simulink model "px4_6dof_quadrotor_bus"  (R2021b)
settings: Solver=VariableStepAuto  StartTime=0.0  StopTime=10.0  FixedStep=plant.motor.dynamic_time_sample/10  RelTol=1e-3
undefined symbols (not defined in the file or in its folder): angular_rate, ax, ay, az, body, controller, DiscIntNeverNeededParam, dphi, dpsi, dtheta, lag, land_detector, lead, magnitude, ned, notch, phi, pitch, plant, psi, rad, roll, s, theta, thrust, vx, vy, vz, w1, w2, w3, w4, x, y, yaw, z
libraries: cstblocks x33, aerolibconvert2 x4, simulink_extras x3, simulink x3, sharedtransform x1
(part 1 of 2)
settings Model: Creator=iftach  LastModifiedBy=iftach
settings SolverCC: ZeroCrossAlgorithm=Adaptive
settings DebuggingCC: MaskedZcDiagnostic=none  IgnoredZcDiagnostic=none

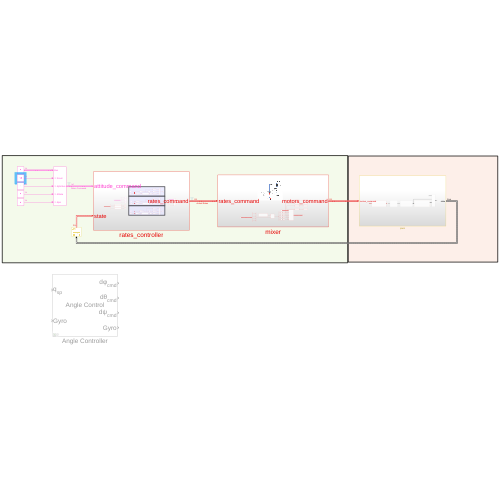
[thumbnail: Simulink's stored preview of the top-level diagram]
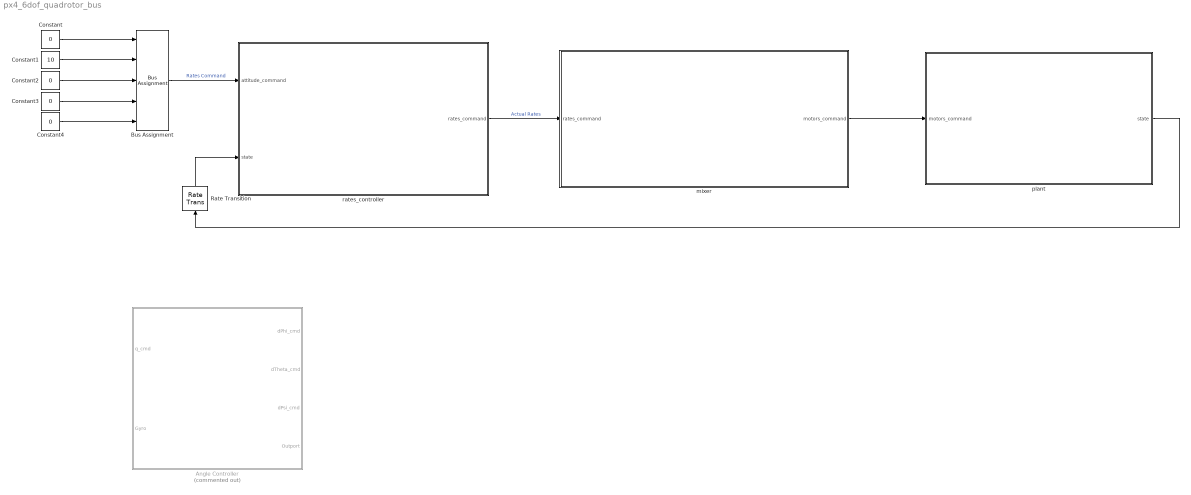
== system px4_6dof_quadrotor_bus ==
  Angle Controller : Subsystem  Commented=on  mask{MC_ROLL_P=4, MC_PITCH_P=4, MC_YAW_P=4, MC_ROLLRATE_MAX=2, MC_PITCHRATE_MAX=2, MC_YAWRATE_MAX=2, MC_ACRO_R_MAX=2, MC_YAW_WEIGHT=0.1, m=0.9}
      mask prompts: MC_ROLL_P "MC_ROLL_P ="; MC_PITCH_P "MC_PITCH_P ="; MC_YAW_P "MC_YAW_P ="; MC_ROLLRATE_MAX "MC_ROLLRATE_MAX ="; MC_PITCHRATE_MAX "MC_PITCHRATE_MAX ="; MC_YAWRATE_MAX "MC_YAWRATE_MAX ="; MC_ACRO_R_MAX "MC_ACRO_R_MAX ="; MC_YAW_WEIGHT "MC_YAW_WEIGHT ="; m "m [kg] ="
      mask DialogControl DescTextVar Prompt: Attitude Controller - based on PX4 architecture
      mask Display:
      | disp('Angle Control')
      | 
      | port_label('input',1,'q_{sp}','texmode','on')
      | port_label('input',2,'Gyro')
      | 
      | port_label('output',1,'d\phi_{cmd}','texmode','on')
      | port_label('output',2,'d\theta_{cmd}','texmode','on')
      | port_label('output',3,'d\psi_{cmd}','texmode','on')
      | port_label('output',4,'Gyro','texmode','on')
  Bus Assignment : BusAssignment  AssignedSignals=thrust,dphi,dtheta,dpsi
  Constant : Constant  Value=0  OutDataTypeStr=Bus: AttitudeCommand
  Constant1 : Constant  Value=10
  Constant2 : Constant  Value=0
  Constant3 : Constant  Value=0
  Constant4 : Constant  Value=0
  Rate Transition : RateTransition  OutPortSampleTime=controller.rate.time_sample
  mixer : Subsystem
  plant : Subsystem
  rates_controller : Subsystem
  wires:
  plant/1(state) -> Rate Transition/1
  mixer/1(motors_command) -> plant/1(motors_command)
  rates_controller/1(rates_command) -> mixer/1(rates_command)  "Actual Rates"
  Rate Transition/1 -> rates_controller/2(state)
  Constant/1 -> Bus Assignment/1
  Bus Assignment/1 -> rates_controller/1(attitude_command)  "Rates Command"
  Constant1/1 -> Bus Assignment/2
  Constant2/1 -> Bus Assignment/3
  Constant3/1 -> Bus Assignment/4
  Constant4/1 -> Bus Assignment/5

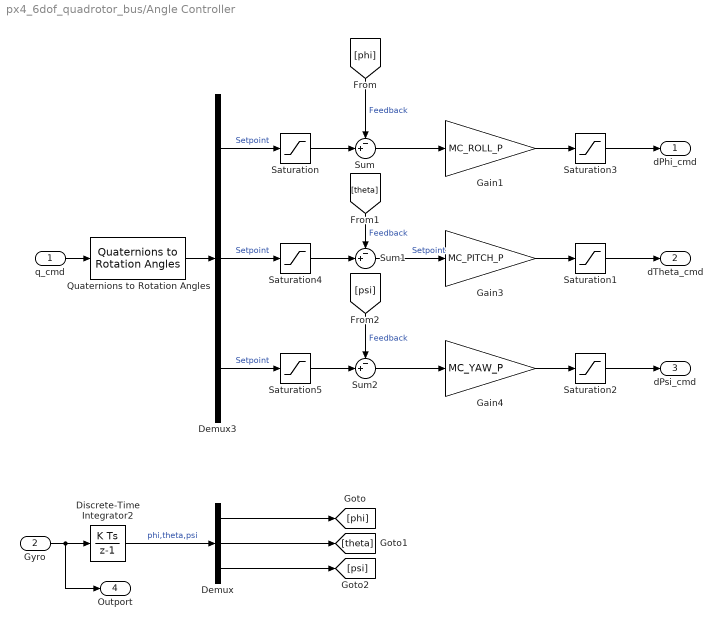
== system px4_6dof_quadrotor_bus/Angle Controller ==
  q_cmd : Inport
  Gyro : Inport  Port=2
  Demux : Demux  Outputs=3
  Demux3 : Demux  Outputs=3
  Discrete-Time Integrator2 : DiscreteIntegrator  InitialCondition=[0.001;0.001;0.001]  SampleTime=-1  ICPrevOutput=DiscIntNeverNeededParam  ICPrevScaledInput=DiscIntNeverNeededParam
  Gain1 : Gain  Gain=MC_ROLL_P
  Gain3 : Gain  Gain=MC_PITCH_P
  Gain4 : Gain  Gain=MC_YAW_P
  Quaternions to Rotation Angles : sharedtransform/Quaternions to Rotation Angles  rotationOrder=XYZ  aMode=aMode
      settings: SourceProductBaseCode=AE,PW,DR,MT,UV,VE
  Saturation : Saturate  UpperLimit=1.5  LowerLimit=-1.5
  Saturation1 : Saturate  UpperLimit=MC_PITCHRATE_MAX  LowerLimit=-MC_PITCHRATE_MAX
  Saturation2 : Saturate  UpperLimit=MC_YAWRATE_MAX  LowerLimit=-MC_YAWRATE_MAX
  Saturation3 : Saturate  UpperLimit=MC_ROLLRATE_MAX  LowerLimit=-MC_ROLLRATE_MAX
  Saturation4 : Saturate  UpperLimit=1.5  LowerLimit=-1.5
  Saturation5 : Saturate  UpperLimit=1.5  LowerLimit=-1.5
  Sum : Sum  Inputs=-+|
  Sum1 : Sum  Inputs=-+|
  Sum2 : Sum  Inputs=-+|
  dPhi_cmd : Outport
  dTheta_cmd : Outport  Port=2
  dPsi_cmd : Outport  Port=3
  Outport : Outport  Port=4
  wires:
  Saturation5/1 -> Sum2/2
  Saturation4/1 -> Sum1/2
  Saturation/1 -> Sum/2
  Quaternions to Rotation Angles/1 -> Demux3/1
  q_cmd/1 -> Quaternions to Rotation Angles/1
  Sum1/1 -> Gain3/1  "Setpoint"
  [psi] -> Sum2/1  "Feedback"
  Sum2/1 -> Gain4/1
  [theta] -> Sum1/1  "Feedback"
  Sum/1 -> Gain1/1
  [phi] -> Sum/1  "Feedback"
  Saturation2/1 -> dPsi_cmd/1
  Saturation1/1 -> dTheta_cmd/1
  Gain4/1 -> Saturation2/1
  Gain3/1 -> Saturation1/1
  Gain1/1 -> Saturation3/1
  Saturation3/1 -> dPhi_cmd/1
  Demux3/3 -> Saturation5/1  "Setpoint"
  Demux3/2 -> Saturation4/1  "Setpoint"
  Demux3/1 -> Saturation/1  "Setpoint"
  Demux/3 -> [psi]
  Demux/1 -> [phi]
  Demux/2 -> [theta]
  Gyro/1 -> Discrete-Time Integrator2/1, Outport/1
  Discrete-Time Integrator2/1 -> Demux/1  "phi,theta,psi"

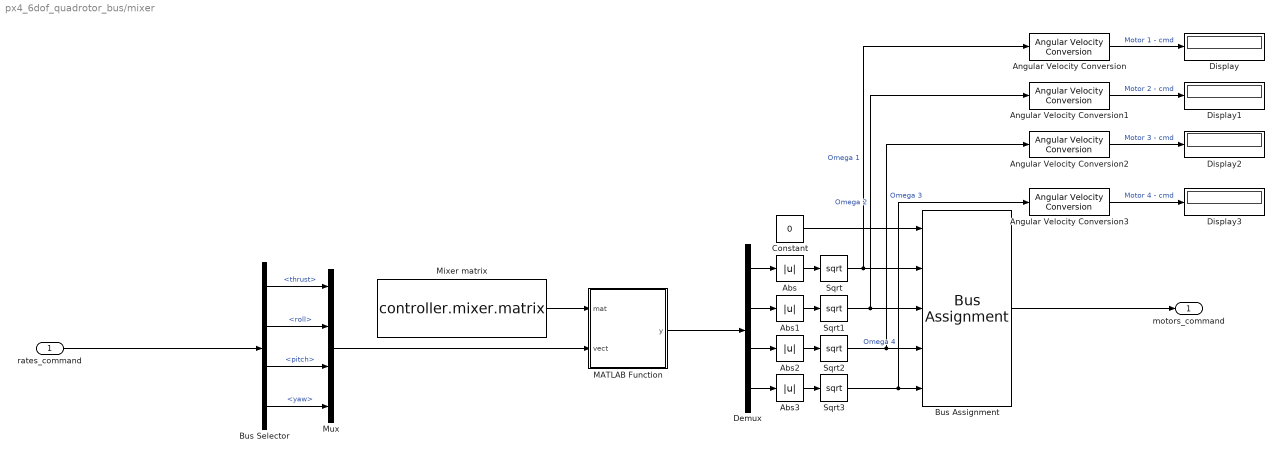
== system px4_6dof_quadrotor_bus/mixer ==
  rates_command : Inport  OutDataTypeStr=Bus: RatesCommand
  Abs{,1..3} (4 alike) : Abs
  Angular Velocity Conversion{,1..3} (4 alike) : aerolibconvert2/Angular Velocity Conversion  IU=rad/s  OU=rpm
  Bus Assignment : BusAssignment  AssignedSignals=w1,w2,w3,w4
  Bus Selector : BusSelector  OutputSignals=thrust,roll,pitch,yaw
  Constant : Constant  Value=0  OutDataTypeStr=Bus: MotorsCommand  SampleTime=controller.rate.time_sample
  Demux : Demux
  Display{,1..3} (4 alike) : Display
  MATLAB Function : MATLAB Function  TreatAsAtomicUnit=on
  Mixer matrix : Constant  StartFcn=|  Value=controller.mixer.matrix  OutDataTypeStr=Inherit: Inherit via back propagation  SampleTime=controller.rate.time_sample
      | %p = Simulink.Mask.get('ControlsModels/Moments and Forces');
      | 
      | Ct = 0.025
      | Cq = 2e-6;
      | 
      | %Ct = p.getParameter('Ct');
      | %Cq =p.getParameter('Cq');
      | 
      | %Ct = str2double(Ct.Value);
      | %Cq = str2double(Cq.Value);
  Mux : Mux
  Sqrt{,1..3} (4 alike) : Sqrt  SaturateOnIntegerOverflow=on
  motors_command : Outport
  wires:
  Demux/1 -> Abs/1
  Demux/2 -> Abs1/1
  Demux/3 -> Abs2/1
  Demux/4 -> Abs3/1
  MATLAB Function/1(y) -> Demux/1
  Mux/1 -> MATLAB Function/2(vect)
  Mixer matrix/1 -> MATLAB Function/1(mat)
  Sqrt/1 -> Bus Assignment/2, Angular Velocity Conversion/1  "Omega 1"
  Sqrt1/1 -> Bus Assignment/3, Angular Velocity Conversion1/1  "Omega 2"
  Sqrt2/1 -> Bus Assignment/4, Angular Velocity Conversion2/1  "Omega 3"
  Sqrt3/1 -> Bus Assignment/5, Angular Velocity Conversion3/1  "Omega 4"
  Angular Velocity Conversion/1 -> Display/1  "Motor 1 - cmd"
  Angular Velocity Conversion1/1 -> Display1/1  "Motor 2 - cmd"
  Angular Velocity Conversion2/1 -> Display2/1  "Motor 3 - cmd"
  Angular Velocity Conversion3/1 -> Display3/1  "Motor 4 - cmd"
  Abs/1 -> Sqrt/1
  Abs1/1 -> Sqrt1/1
  Abs2/1 -> Sqrt2/1
  Abs3/1 -> Sqrt3/1
  Constant/1 -> Bus Assignment/1
  Bus Assignment/1 -> motors_command/1
  rates_command/1 -> Bus Selector/1
  Bus Selector/1 -> Mux/1  "<thrust>"
  Bus Selector/2 -> Mux/2  "<roll>"
  Bus Selector/3 -> Mux/3  "<pitch>"
  Bus Selector/4 -> Mux/4  "<yaw>"

== system px4_6dof_quadrotor_bus/plant ==
  motors_command : Inport  OutDataTypeStr=Bus: MotorsCommand
  Bus Assignment : BusAssignment  AssignedSignals=body,ned,land_detector
  Constant : Constant  Value=0  OutDataTypeStr=Bus: PlantState  SampleTime=-1
  Rate Transition : RateTransition  OutPortSampleTime=0
  Rate Transition1 : RateTransition  OutPortSampleTime=0
  angle2body : Subsystem
  body2ned : Subsystem
  control2motors : Subsystem
  motors2angles : Subsystem
  state : Outport  OutDataTypeStr=Bus: PlantState
  wires:
  motors_command/1 -> control2motors/1(controller_command)
  control2motors/1(motors_velocities) -> Rate Transition/1  "Motors"
  motors2angles/1(angles) -> angle2body/1(angles)  "Body"
  angle2body/1(body) -> Bus Assignment/2, body2ned/1(body)
  Constant/1 -> Bus Assignment/1
  body2ned/1(NED) -> Bus Assignment/3
  Bus Assignment/1 -> state/1  "State"
  Rate Transition/1 -> motors2angles/1(motors_velocities)
  body2ned/2(land_detector) -> Rate Transition1/1
  Rate Transition1/1 -> Bus Assignment/4

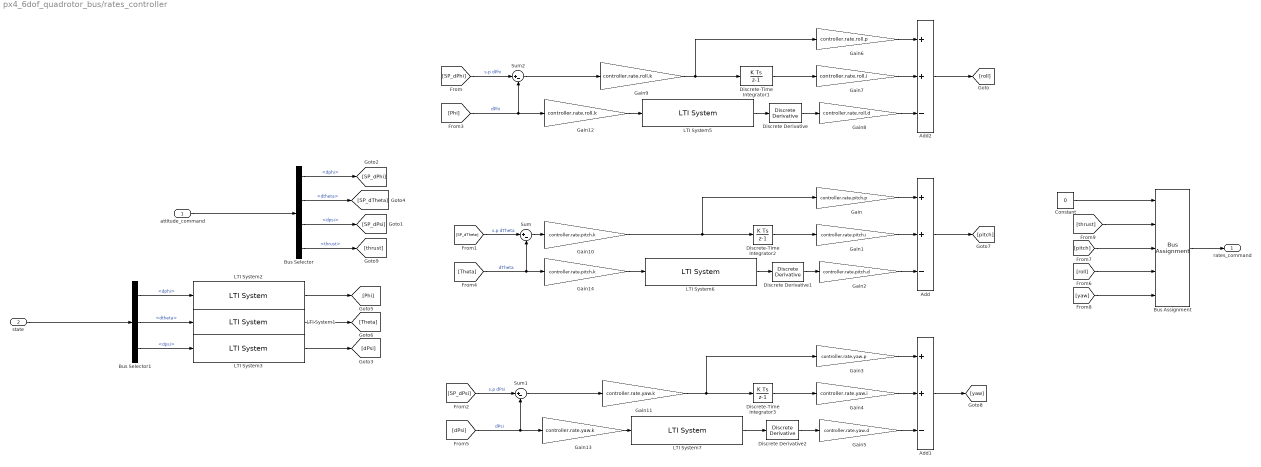
== system px4_6dof_quadrotor_bus/rates_controller ==
  attitude_command : Inport  OutDataTypeStr=Bus: AttitudeCommand
  state : Inport  Port=2  OutDataTypeStr=Bus: PlantState
  Add : Sum  Inputs=++-
  Add1 : Sum  Inputs=++-
  Add2 : Sum  Inputs=++-
  Bus Assignment : BusAssignment  AssignedSignals=thrust,pitch,roll,yaw
  Bus Selector : BusSelector  OutputSignals=dphi,dtheta,dpsi,thrust
  Bus Selector1 : BusSelector  OutputSignals=body.dphi,body.dtheta,body.dpsi
  Constant : Constant  Value=0  OutDataTypeStr=Bus: RatesCommand
  Discrete Derivative : simulink/Discrete/Discrete Derivative  gainval=1.0  ICPrevScaledInput=0.0  OutMin=[]  OutMax=[]  OutDataType=fixdt(1, 16)  OutScaling=2^-10  DoSatur=off
  Discrete Derivative1 : simulink/Discrete/Discrete Derivative  gainval=1.0  ICPrevScaledInput=0.0  OutMin=[]  OutMax=[]  OutDataType=fixdt(1, 16)  OutScaling=2^-10  DoSatur=off
  Discrete Derivative2 : simulink/Discrete/Discrete Derivative  gainval=1.0  ICPrevScaledInput=0.0  OutMin=[]  OutMax=[]  OutDataType=fixdt(1, 16)  OutScaling=2^-10  DoSatur=off
  Discrete-Time Integrator1 : DiscreteIntegrator  SampleTime=controller.rate.time_sample  LimitOutput=on  UpperSaturationLimit=controller.rate.mc_rr_int_limit  LowerSaturationLimit=-controller.rate.mc_rr_int_limit  ICPrevOutput=DiscIntNeverNeededParam  ICPrevScaledInput=DiscIntNeverNeededParam
  Discrete-Time Integrator2 : DiscreteIntegrator  SampleTime=controller.rate.time_sample  LimitOutput=on  UpperSaturationLimit=controller.rate.mc_pr_int_limit  LowerSaturationLimit=-controller.rate.mc_pr_int_limit  ICPrevOutput=DiscIntNeverNeededParam  ICPrevScaledInput=DiscIntNeverNeededParam
  Discrete-Time Integrator3 : DiscreteIntegrator  SampleTime=controller.rate.time_sample  LimitOutput=on  UpperSaturationLimit=controller.rate.mc_yr_int_limit  LowerSaturationLimit=-controller.rate.mc_yr_int_limit  ICPrevOutput=DiscIntNeverNeededParam  ICPrevScaledInput=DiscIntNeverNeededParam
  Gain : Gain  Gain=controller.rate.pitch.p
  Gain1 : Gain  Gain=controller.rate.pitch.i
  Gain10 : Gain  Gain=controller.rate.pitch.k
  Gain11 : Gain  Gain=controller.rate.yaw.k
  Gain12 : Gain  Gain=controller.rate.roll.k
  Gain13 : Gain  Gain=controller.rate.yaw.k
  Gain14 : Gain  Gain=controller.rate.pitch.k
  Gain2 : Gain  Gain=controller.rate.pitch.d
  Gain3 : Gain  Gain=controller.rate.yaw.p
  Gain4 : Gain  Gain=controller.rate.yaw.i
  Gain5 : Gain  Gain=controller.rate.yaw.d
  Gain6 : Gain  Gain=controller.rate.roll.p
  Gain7 : Gain  Gain=controller.rate.roll.i
  Gain8 : Gain  Gain=controller.rate.roll.d
  Gain9 : Gain  Gain=controller.rate.roll.k
  LTI System1 : cstblocks/LTI System  sys=c2d(tf(1,[controller.filters.gyro_cutoff 1]),controller.rate.time_sample)  IC=[]
  LTI System2 : cstblocks/LTI System  sys=c2d(tf(1,[controller.filters.gyro_cutoff 1]),controller.rate.time_sample)  IC=[]
  LTI System3 : cstblocks/LTI System  sys=c2d(tf(1,[controller.filters.gyro_cutoff 1]),controller.rate.time_sample)  IC=[]
  LTI System5 : cstblocks/LTI System  sys=c2d(tf(1,[controller.filters.dgyro_cutoff 1]),controller.rate.time_sample)  IC=[]
  LTI System6 : cstblocks/LTI System  sys=c2d(tf(1,[controller.filters.dgyro_cutoff 1]),controller.rate.time_sample)  IC=[]
  LTI System7 : cstblocks/LTI System  sys=c2d(tf(1,[controller.filters.dgyro_cutoff 1]),controller.rate.time_sample)  IC=[]
  Sum : Sum  Inputs=|+-
  Sum1 : Sum  Inputs=|+-
  Sum2 : Sum  Inputs=|+-
  rates_command : Outport  OutDataTypeStr=Bus: RatesCommand
  wires:
  Bus Selector/2 -> [SP_dTheta]  "<dtheta>"
  LTI System6/1 -> Discrete Derivative1/1
  Sum/1 -> Gain10/1
  Discrete-Time Integrator2/1 -> Gain1/1
  Gain2/1 -> Add/3
  Gain1/1 -> Add/2
  Gain/1 -> Add/1
  Gain3/1 -> Add1/1
  Gain4/1 -> Add1/2
  Gain5/1 -> Add1/3
  Discrete-Time Integrator3/1 -> Gain4/1
  Sum1/1 -> Gain11/1
  LTI System7/1 -> Discrete Derivative2/1
  [dPsi] -> Gain13/1, Sum1/2  "dPsi"
  [SP_dPsi] -> Sum1/1  "s.p dPsi"
  Add/1 -> [pitch]
  Bus Assignment/1 -> rates_command/1
  Gain6/1 -> Add2/1
  Gain7/1 -> Add2/2
  Gain8/1 -> Add2/3
  Discrete-Time Integrator1/1 -> Gain7/1
  Sum2/1 -> Gain9/1
  LTI System5/1 -> Discrete Derivative/1
  [SP_dPhi] -> Sum2/1  "s.p dPhi"
  [SP_dTheta] -> Sum/1  "s.p dTheta"
  [Phi] -> Gain12/1, Sum2/2  "dPhi"
  [Theta] -> Gain14/1, Sum/2  "dTheta"
  Add2/1 -> [roll]
  Add1/1 -> [yaw]
  Discrete Derivative/1 -> Gain8/1
  Discrete Derivative1/1 -> Gain2/1
  Discrete Derivative2/1 -> Gain5/1
  Gain9/1 -> Discrete-Time Integrator1/1, Gain6/1
  Gain10/1 -> Discrete-Time Integrator2/1, Gain/1
  Gain11/1 -> Discrete-Time Integrator3/1, Gain3/1
  Gain12/1 -> LTI System5/1
  Gain13/1 -> LTI System7/1
  Gain14/1 -> LTI System6/1
  state/1 -> Bus Selector1/1
  Bus Selector1/3 -> LTI System3/1  "<dpsi>"
  LTI System2/1 -> [Phi]
  LTI System1/1 -> [Theta]
  LTI System3/1 -> [dPsi]
  Bus Selector/3 -> [SP_dPsi]  "<dpsi>"
  Bus Selector/1 -> [SP_dPhi]  "<dphi>"
  attitude_command/1 -> Bus Selector/1
  Bus Selector1/1 -> LTI System2/1  "<dphi>"
  Bus Selector1/2 -> LTI System1/1  "<dtheta>"
  Constant/1 -> Bus Assignment/1
  [roll] -> Bus Assignment/4
  [pitch] -> Bus Assignment/3
  [yaw] -> Bus Assignment/5
  Bus Selector/4 -> [thrust]  "<thrust>"
  [thrust] -> Bus Assignment/2

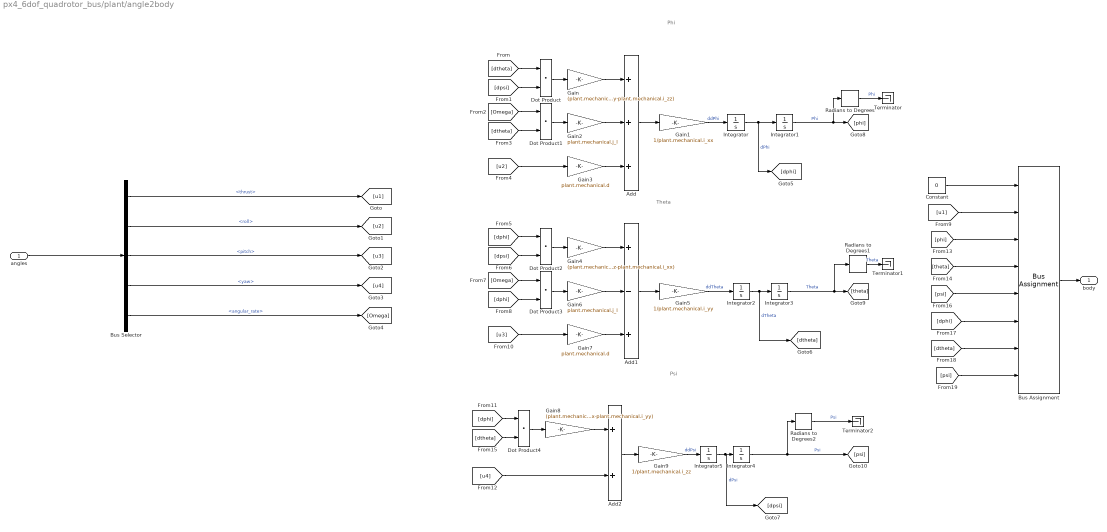
== system px4_6dof_quadrotor_bus/plant/angle2body ==
  note: Phi
  note: Theta
  note: Psi
  angles : Inport  OutDataTypeStr=Bus: PlantAngles
  Add : Sum  Inputs=3
  Add1 : Sum  Inputs=+-+
  Add2 : Sum  Inputs=2
  Bus Assignment : BusAssignment  AssignedSignals=thrust,phi,theta,psi,dphi,dtheta,dpsi
  Bus Selector : BusSelector  OutputSignals=thrust,roll,pitch,yaw,angular_rate
  Constant : Constant  Value=0  OutDataTypeStr=Bus: PlantBody  SampleTime=-1
  Dot Product{,1..4} (5 alike) : DotProduct  InputSameDT=on  OutDataTypeStr=Inherit: Inherit via internal rule
  Gain : Gain  Gain=(plant.mechanical.i_yy-plant.mechanical.i_zz)
  Gain1 : Gain  Gain=1/plant.mechanical.i_xx
  Gain2 : Gain  Gain=plant.mechanical.j_l
  Gain3 : Gain  Gain=plant.mechanical.d
  Gain4 : Gain  Gain=(plant.mechanical.i_zz-plant.mechanical.i_xx)
  Gain5 : Gain  Gain=1/plant.mechanical.i_yy
  Gain6 : Gain  Gain=plant.mechanical.j_l
  Gain7 : Gain  Gain=plant.mechanical.d
  Gain8 : Gain  Gain=(plant.mechanical.i_xx-plant.mechanical.i_yy)
  Gain9 : Gain  Gain=1/plant.mechanical.i_zz
  Integrator{,1..5} (6 alike) : Integrator
  Radians to Degrees : simulink_extras/Transformations/Radians to Degrees
  Radians to Degrees1 : simulink_extras/Transformations/Radians to Degrees
  Radians to Degrees2 : simulink_extras/Transformations/Radians to Degrees
  Terminator : Terminator
  Terminator1 : Terminator
  Terminator2 : Terminator
  body : Outport  OutDataTypeStr=Bus: PlantBody
  wires:
  Integrator/1 -> [dphi], Integrator1/1  "dPhi"
  Integrator2/1 -> Integrator3/1, [dtheta]  "dTheta"
  Integrator5/1 -> [dpsi], Integrator4/1  "dPsi"
  Integrator1/1 -> [phi], Radians to Degrees/1  "Phi"
  Integrator3/1 -> Radians to Degrees1/1, [theta]  "Theta"
  Integrator4/1 -> Radians to Degrees2/1, [psi]  "Psi"
  [dpsi] -> Dot Product/2
  [dtheta] -> Dot Product/1
  Dot Product/1 -> Gain/1
  Gain/1 -> Add/1
  Gain1/1 -> Integrator/1  "ddPhi"
  Add/1 -> Gain1/1
  [Omega] -> Dot Product1/1
  Dot Product1/1 -> Gain2/1
  [dtheta] -> Dot Product1/2
  Gain2/1 -> Add/2
  [u2] -> Gain3/1
  Gain7/1 -> Add1/3
  [u3] -> Gain7/1
  Gain6/1 -> Add1/2
  [dphi] -> Dot Product3/2
  Dot Product3/1 -> Gain6/1
  [Omega] -> Dot Product3/1
  Add1/1 -> Gain5/1
  Gain4/1 -> Add1/1
  Dot Product2/1 -> Gain4/1
  [dphi] -> Dot Product2/1
  [dpsi] -> Dot Product2/2
  Gain5/1 -> Integrator2/1  "ddTheta"
  [dtheta] -> Dot Product4/2
  Dot Product4/1 -> Gain8/1
  Gain8/1 -> Add2/1
  Add2/1 -> Gain9/1
  Gain9/1 -> Integrator5/1  "ddPsi"
  [dphi] -> Dot Product4/1
  [u4] -> Add2/2
  Gain3/1 -> Add/3
  Radians to Degrees/1 -> Terminator/1  "Phi"
  Radians to Degrees1/1 -> Terminator1/1  "Theta"
  Radians to Degrees2/1 -> Terminator2/1  "Psi"
  Bus Selector/1 -> [u1]  "<thrust>"
  Bus Selector/2 -> [u2]  "<roll>"
  Bus Selector/3 -> [u3]  "<pitch>"
  Bus Selector/4 -> [u4]  "<yaw>"
  Bus Selector/5 -> [Omega]  "<angular_rate>"
  Bus Assignment/1 -> body/1
  Constant/1 -> Bus Assignment/1
  [u1] -> Bus Assignment/2
  [phi] -> Bus Assignment/3
  [theta] -> Bus Assignment/4
  [psi] -> Bus Assignment/5
  [dphi] -> Bus Assignment/6
  [dtheta] -> Bus Assignment/7
  [psi] -> Bus Assignment/8
  angles/1 -> Bus Selector/1

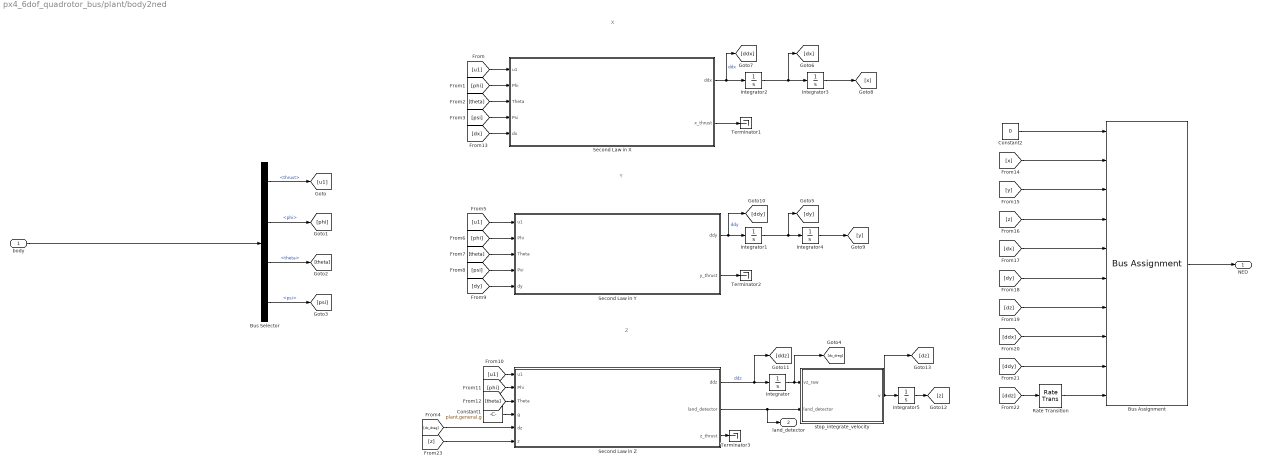
== system px4_6dof_quadrotor_bus/plant/body2ned ==
  note: X
  note: Y
  note: Z
  body : Inport  OutDataTypeStr=Bus: PlantBody
  Bus Assignment : BusAssignment  AssignedSignals=x,y,z,vx,vy,vz,ax,ay,az
  Bus Selector : BusSelector  OutputSignals=thrust,phi,theta,psi
  Constant1 : Constant  Value=plant.general.g  SampleTime=-1
  Constant2 : Constant  Value=0  OutDataTypeStr=Bus: PlantNed
  Integrator : Integrator  InitialCondition=plant.ic.velocity.z
  Integrator1 : Integrator  InitialCondition=plant.ic.velocity.y
  Integrator2 : Integrator  InitialCondition=plant.ic.velocity.x
  Integrator3 : Integrator  InitialCondition=plant.ic.position.x
  Integrator4 : Integrator  InitialCondition=plant.ic.position.y
  Integrator5 : Integrator  InitialCondition=plant.ic.position.z  LimitOutput=on  UpperSaturationLimit=0
  Rate Transition : RateTransition  OutPortSampleTime=0
  Second Law in X : Subsystem
  Second Law in Y : Subsystem
  Second Law in Z : Subsystem
  Terminator1 : Terminator
  Terminator2 : Terminator
  Terminator3 : Terminator
  stop_integrate_velocity : MATLAB Function  TreatAsAtomicUnit=on
  NED : Outport  OutDataTypeStr=Bus: PlantNed
  land_detector : Outport  Port=2  OutDataTypeStr=boolean
  wires:
  Second Law in X/1(ddx) -> [ddx], Integrator2/1  "ddx"
  [u1] -> Second Law in X/1(u1)
  [phi] -> Second Law in X/2(Phi)
  [theta] -> Second Law in X/3(Theta)
  [psi] -> Second Law in X/4(Psi)
  [psi] -> Second Law in Y/4(Psi)
  [theta] -> Second Law in Y/3(Theta)
  [phi] -> Second Law in Y/2(Phi)
  [u1] -> Second Law in Y/1(u1)
  Second Law in Y/1(ddy) -> [ddy], Integrator1/1  "ddy"
  Second Law in Z/1(ddz) -> Integrator/1, [ddz]  "ddz"
  [u1] -> Second Law in Z/1(u1)
  [phi] -> Second Law in Z/2(Phi)
  [theta] -> Second Law in Z/3(Theta)
  Constant1/1 -> Second Law in Z/4(g)
  [dy] -> Second Law in Y/5(dy)
  [dx] -> Second Law in X/5(dx)
  Integrator2/1 -> Integrator3/1, [dx]
  Integrator1/1 -> Integrator4/1, [dy]
  body/1 -> Bus Selector/1
  Bus Selector/1 -> [u1]  "<thrust>"
  Bus Selector/2 -> [phi]  "<phi>"
  Bus Selector/3 -> [theta]  "<theta>"
  Bus Selector/4 -> [psi]  "<psi>"
  Integrator3/1 -> [x]
  Integrator4/1 -> [y]
  Constant2/1 -> Bus Assignment/1
  [x] -> Bus Assignment/2
  [y] -> Bus Assignment/3
  [z] -> Bus Assignment/4
  [dx] -> Bus Assignment/5
  [dy] -> Bus Assignment/6
  [dz] -> Bus Assignment/7
  [ddx] -> Bus Assignment/8
  [ddy] -> Bus Assignment/9
  [ddz] -> Rate Transition/1
  Bus Assignment/1 -> NED/1
  Second Law in X/2(x_thrust) -> Terminator1/1
  Second Law in Y/2(y_thrust) -> Terminator2/1
  Second Law in Z/3(z_thrust) -> Terminator3/1
  Integrator5/1 -> [z]
  [dz_drag] -> Second Law in Z/5(dz)
  Second Law in Z/2(land_detector) -> land_detector/1, stop_integrate_velocity/2(land_detector)
  [z] -> Second Law in Z/6(z)
  Integrator/1 -> [dz_drag], stop_integrate_velocity/1(vz_raw)
  Rate Transition/1 -> Bus Assignment/10
  stop_integrate_velocity/1(v) -> [dz], Integrator5/1

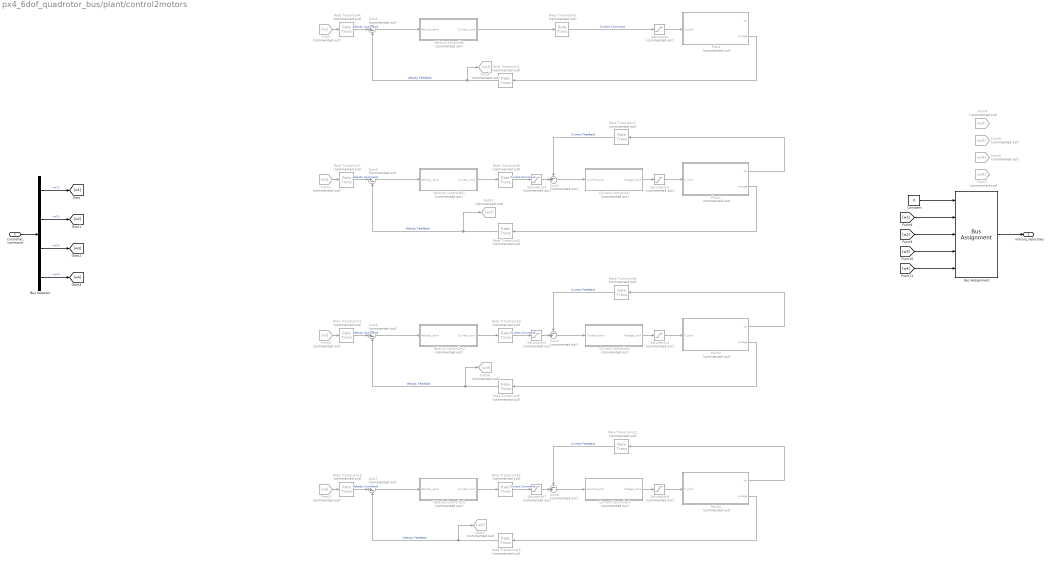
== system px4_6dof_quadrotor_bus/plant/control2motors ==
  controller_command : Inport  OutDataTypeStr=Bus: MotorsCommand
  Bus Assignment : BusAssignment  AssignedSignals=w1,w2,w3,w4
  Bus Selector : BusSelector  OutputSignals=w1,w2,w3,w4
  Constant : Constant  Value=0  OutDataTypeStr=Bus: PlantMotorsVelocity
  Current Controller1 : Subsystem  Commented=on
  Current Controller2 : Subsystem  Commented=on
  Current Controller3 : Subsystem  Commented=on
  From : From  Commented=on  GotoTag=w1
  From1 : From  Commented=on  GotoTag=w2
  From2 : From  Commented=on  GotoTag=w3
  From3 : From  Commented=on  GotoTag=w4
  From4 : From  Commented=on  GotoTag=w1f
  From5 : From  Commented=on  GotoTag=w2f
  From6 : From  Commented=on  GotoTag=w3f
  From7 : From  Commented=on  GotoTag=w4f
  Goto4 : Goto  Commented=on  GotoTag=w1f
  Goto5 : Goto  Commented=on  GotoTag=w2f
  Goto6 : Goto  Commented=on  GotoTag=w3f
  Goto7 : Goto  Commented=on  GotoTag=w4f
  Plant : Subsystem  Commented=on
  Plant1 : Subsystem  Commented=on
  Plant2 : Subsystem  Commented=on
  Plant3 : Subsystem  Commented=on
  Rate Transition{1,3,6,8,10,12,14} (7 alike) : RateTransition  Commented=on  OutPortSampleTime=plant.motor.electric_time_sample
  Rate Transition{2,4..5,7,9,11,13,15} (8 alike) : RateTransition  Commented=on  OutPortSampleTime=plant.motor.dynamic_time_sample
  Saturation{,1,4,6} (4 alike) : Saturate  Commented=on  UpperLimit=plant.motor.max_v  LowerLimit=-plant.motor.max_v
  Saturation3 : Saturate  Commented=on  UpperLimit=plant.motor.max_i  LowerLimit=-plant.motor.max_i
  Saturation5 : Saturate  Commented=on  UpperLimit=plant.motor.max_i  LowerLimit=-plant.motor.max_i
  Saturation7 : Saturate  Commented=on  UpperLimit=plant.motor.max_i  LowerLimit=-plant.motor.max_i
  Sum{1,3,5,7} (4 alike) : Sum  Commented=on  Inputs=|+-
  Sum2 : Sum  Commented=on  Inputs=-+|
  Sum4 : Sum  Commented=on  Inputs=-+|
  Sum6 : Sum  Commented=on  Inputs=-+|
  Velocity Controller : Subsystem  Commented=on
  Velocity Controller1 : Subsystem  Commented=on
  Velocity Controller2 : Subsystem  Commented=on
  Velocity Controller3 : Subsystem  Commented=on
  motors_velocities : Outport  OutDataTypeStr=Bus: PlantMotorsVelocity
  wires:
  Saturation/1 -> Plant/1(V_cmd)
  Velocity Controller/1(Current_cmd) -> Rate Transition3/1
  Rate Transition3/1 -> Saturation/1  "Current Command"
  Rate Transition2/1 -> Goto4/1, Sum1/2  "Velocity Feedback"
  Plant/2(omega) -> Rate Transition2/1
  Sum1/1 -> Velocity Controller/1(Velocity_error)
  Rate Transition4/1 -> Sum1/1  "Velocity Command"
  Rate Transition7/1 -> Sum3/1  "Velocity Command"
  Sum2/1 -> Current Controller1/1(Current_error)
  Saturation1/1 -> Plant1/1(V_cmd)
  Rate Transition1/1 -> Sum2/1  "Current Feedback"
  Sum3/1 -> Velocity Controller1/1(Velocity_error)
  Current Controller1/1(Voltage_cmd) -> Saturation1/1
  Plant1/2(omega) -> Rate Transition5/1
  Saturation3/1 -> Sum2/2
  Plant1/1(Im) -> Rate Transition1/1
  Rate Transition5/1 -> Goto5/1, Sum3/2  "Velocity Feedback"
  Rate Transition6/1 -> Saturation3/1  "Current Command"
  Velocity Controller1/1(Current_cmd) -> Rate Transition6/1
  Rate Transition11/1 -> Sum5/1  "Velocity Command"
  Sum4/1 -> Current Controller2/1(Current_error)
  Saturation4/1 -> Plant2/1(V_cmd)
  Rate Transition8/1 -> Sum4/1  "Current Feedback"
  Sum5/1 -> Velocity Controller2/1(Velocity_error)
  Current Controller2/1(Voltage_cmd) -> Saturation4/1
  Plant2/2(omega) -> Rate Transition9/1
  Saturation5/1 -> Sum4/2
  Plant2/1(Im) -> Rate Transition8/1
  Rate Transition9/1 -> Goto6/1, Sum5/2  "Velocity Feedback"
  Rate Transition10/1 -> Saturation5/1  "Current Command"
  Velocity Controller2/1(Current_cmd) -> Rate Transition10/1
  Rate Transition15/1 -> Sum7/1  "Velocity Command"
  Sum6/1 -> Current Controller3/1(Current_error)
  Saturation6/1 -> Plant3/1(V_cmd)
  Rate Transition12/1 -> Sum6/1  "Current Feedback"
  Sum7/1 -> Velocity Controller3/1(Velocity_error)
  Current Controller3/1(Voltage_cmd) -> Saturation6/1
  Plant3/2(omega) -> Rate Transition13/1
  Saturation7/1 -> Sum6/2
  Plant3/1(Im) -> Rate Transition12/1
  Rate Transition13/1 -> Goto7/1, Sum7/2  "Velocity Feedback"
  Rate Transition14/1 -> Saturation7/1  "Current Command"
  Velocity Controller3/1(Current_cmd) -> Rate Transition14/1
  controller_command/1 -> Bus Selector/1
  Bus Selector/1 -> [w1]  "<w1>"
  Bus Selector/2 -> [w2]  "<w2>"
  Bus Selector/3 -> [w3]  "<w3>"
  Bus Selector/4 -> [w4]  "<w4>"
  From/1 -> Rate Transition4/1
  From1/1 -> Rate Transition7/1
  From2/1 -> Rate Transition11/1
  From3/1 -> Rate Transition15/1
  Constant/1 -> Bus Assignment/1
  [w1] -> Bus Assignment/2
  [w2] -> Bus Assignment/3
  [w3] -> Bus Assignment/4
  [w4] -> Bus Assignment/5
  Bus Assignment/1 -> motors_velocities/1

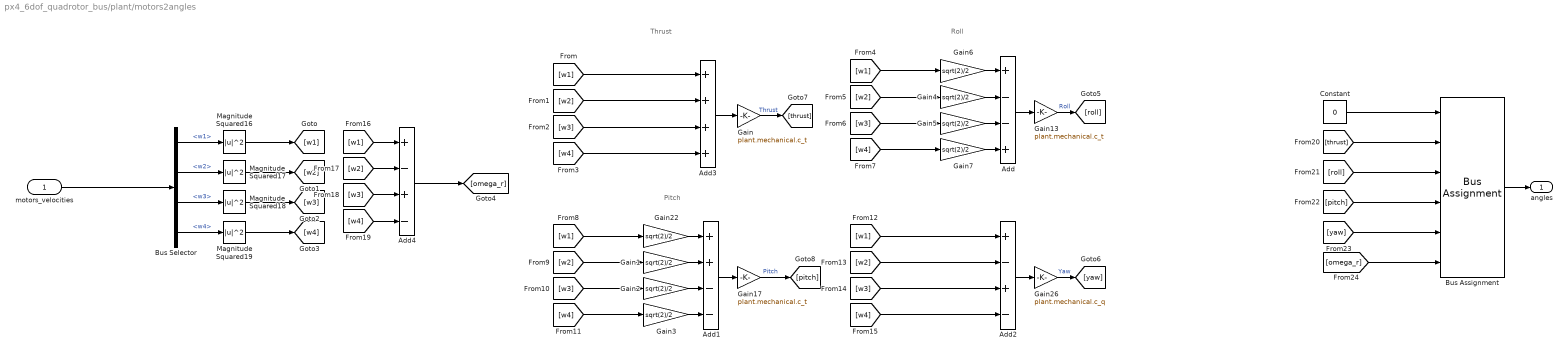
== system px4_6dof_quadrotor_bus/plant/motors2angles ==
  note: Thrust
  note: Roll
  note: Pitch
  motors_velocities : Inport  OutDataTypeStr=Bus: PlantMotorsVelocity
  Add : Sum  Inputs=+--+
  Add1 : Sum  Inputs=++--
  Add2 : Sum  Inputs=+-+-
  Add3 : Sum  Inputs=4
  Add4 : Sum  Inputs=+-+-
  Bus Assignment : BusAssignment  AssignedSignals=thrust,roll,pitch,yaw,angular_rate
  Bus Selector : BusSelector  OutputSignals=w1,w2,w3,w4
  Constant : Constant  Value=0  OutDataTypeStr=Bus: PlantAngles
  Gain : Gain  Gain=plant.mechanical.c_t
  Gain{1..7,22} (8 alike) : Gain  Gain=sqrt(2)/2
  Gain13 : Gain  Gain=plant.mechanical.c_t
  Gain17 : Gain  Gain=plant.mechanical.c_t
  Gain26 : Gain  Gain=plant.mechanical.c_q
  Magnitude Squared{16..19} (4 alike) : Math  Operator=magnitude^2  SaturateOnIntegerOverflow=on
  angles : Outport  OutDataTypeStr=Bus: PlantAngles
  wires:
  [w2] -> Gain4/1
  Gain/1 -> [thrust]  "Thrust"
  Gain1/1 -> Add1/2
  [w3] -> Add2/3
  [w3] -> Gain5/1
  [w3] -> Gain2/1
  Gain22/1 -> Add1/1
  Gain6/1 -> Add/1
  [w1] -> Gain6/1
  Gain2/1 -> Add1/3
  [w4] -> Add2/4
  [w1] -> Gain22/1
  Bus Selector/1 -> Magnitude Squared16/1  "<w1>"
  Bus Selector/2 -> Magnitude Squared17/1  "<w2>"
  Gain13/1 -> [roll]  "Roll"
  Add1/1 -> Gain17/1
  [w1] -> Add2/1
  [w3] -> Add3/3
  [w2] -> Add3/2
  [w2] -> Add4/2
  Gain4/1 -> Add/2
  Bus Selector/4 -> Magnitude Squared19/1  "<w4>"
  Gain26/1 -> [yaw]  "Yaw"
  [w4] -> Gain7/1
  [w2] -> Add2/2
  Bus Selector/3 -> Magnitude Squared18/1  "<w3>"
  Gain3/1 -> Add1/4
  Add/1 -> Gain13/1
  Add3/1 -> Gain/1
  Add2/1 -> Gain26/1
  [w4] -> Add4/4
  [w4] -> Add3/4
  [w1] -> Add3/1
  [w2] -> Gain1/1
  [w4] -> Gain3/1
  Gain5/1 -> Add/3
  Gain7/1 -> Add/4
  [w1] -> Add4/1
  [w3] -> Add4/3
  Gain17/1 -> [pitch]  "Pitch"
  Add4/1 -> [omega_r]
  Bus Assignment/1 -> angles/1
  Constant/1 -> Bus Assignment/1
  motors_velocities/1 -> Bus Selector/1
  [thrust] -> Bus Assignment/2
  [roll] -> Bus Assignment/3
  [pitch] -> Bus Assignment/4
  [yaw] -> Bus Assignment/5
  [omega_r] -> Bus Assignment/6
  Magnitude Squared16/1 -> [w1]
  Magnitude Squared17/1 -> [w2]
  Magnitude Squared18/1 -> [w3]
  Magnitude Squared19/1 -> [w4]

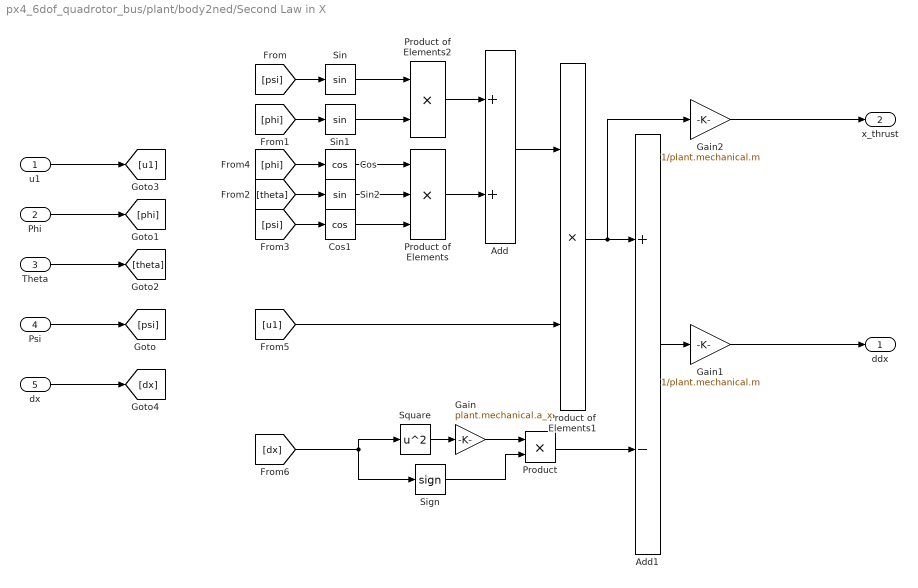
== system px4_6dof_quadrotor_bus/plant/body2ned/Second Law in X ==
  u1 : Inport
  Phi : Inport  Port=2
  Theta : Inport  Port=3
  Psi : Inport  Port=4
  dx : Inport  Port=5
  Add : Sum
  Add1 : Sum  Inputs=+-
  Cos : Trigonometry  Operator=cos
  Cos1 : Trigonometry  Operator=cos
  Gain : Gain  Gain=plant.mechanical.a_x
  Gain1 : Gain  Gain=1/plant.mechanical.m
  Gain2 : Gain  Gain=1/plant.mechanical.m
  Product : Product
  Product of Elements : Product  Inputs=3
  Product of Elements1 : Product
  Product of Elements2 : Product
  Sign : Signum
  Sin : Trigonometry
  Sin1 : Trigonometry
  Sin2 : Trigonometry
  Square : Math  Operator=square  SaturateOnIntegerOverflow=on
  ddx : Outport
  x_thrust : Outport  Port=2
  wires:
  Cos/1 -> Product of Elements/1
  [phi] -> Cos/1
  [psi] -> Cos1/1
  Cos1/1 -> Product of Elements/3
  Sin1/1 -> Product of Elements2/2
  [u1] -> Product of Elements1/2
  Product of Elements/1 -> Add/2
  Product of Elements1/1 -> Gain2/1, Add1/1
  Add/1 -> Product of Elements1/1
  [theta] -> Sin2/1
  Sin2/1 -> Product of Elements/2
  Product of Elements2/1 -> Add/1
  [psi] -> Sin/1
  Sin/1 -> Product of Elements2/1
  [phi] -> Sin1/1
  Add1/1 -> Gain1/1
  Psi/1 -> [psi]
  Phi/1 -> [phi]
  Theta/1 -> [theta]
  u1/1 -> [u1]
  dx/1 -> [dx]
  Gain1/1 -> ddx/1
  Square/1 -> Gain/1
  [dx] -> Square/1, Sign/1
  Gain/1 -> Product/1
  Sign/1 -> Product/2
  Product/1 -> Add1/2
  Gain2/1 -> x_thrust/1

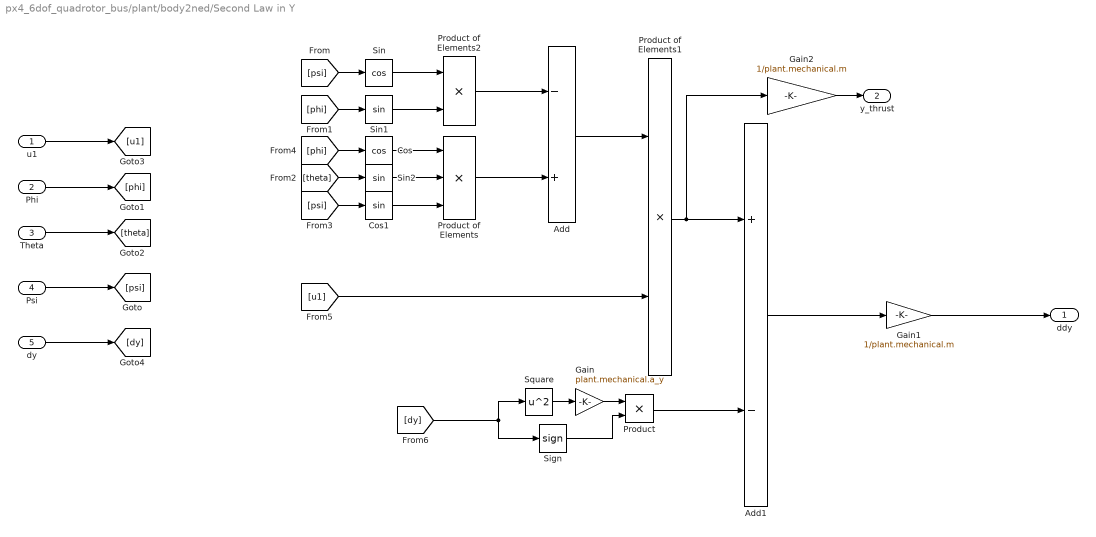
== system px4_6dof_quadrotor_bus/plant/body2ned/Second Law in Y ==
  u1 : Inport
  Phi : Inport  Port=2
  Theta : Inport  Port=3
  Psi : Inport  Port=4
  dy : Inport  Port=5
  Add : Sum  Inputs=-+
  Add1 : Sum  Inputs=+-
  Cos : Trigonometry  Operator=cos
  Cos1 : Trigonometry
  Gain : Gain  Gain=plant.mechanical.a_y
  Gain1 : Gain  Gain=1/plant.mechanical.m
  Gain2 : Gain  Gain=1/plant.mechanical.m
  Product : Product
  Product of Elements : Product  Inputs=3
  Product of Elements1 : Product
  Product of Elements2 : Product
  Sign : Signum
  Sin : Trigonometry  Operator=cos
  Sin1 : Trigonometry
  Sin2 : Trigonometry
  Square : Math  Operator=square  SaturateOnIntegerOverflow=on
  ddy : Outport
  y_thrust : Outport  Port=2
  wires:
  dy/1 -> [dy]
  u1/1 -> [u1]
  Theta/1 -> [theta]
  Phi/1 -> [phi]
  Psi/1 -> [psi]
  Add1/1 -> Gain1/1
  [phi] -> Sin1/1
  Sin/1 -> Product of Elements2/1
  [psi] -> Sin/1
  Product of Elements2/1 -> Add/1
  Sin2/1 -> Product of Elements/2
  [theta] -> Sin2/1
  Add/1 -> Product of Elements1/1
  Product of Elements1/1 -> Gain2/1, Add1/1
  Product of Elements/1 -> Add/2
  [u1] -> Product of Elements1/2
  Sin1/1 -> Product of Elements2/2
  Cos1/1 -> Product of Elements/3
  [psi] -> Cos1/1
  [phi] -> Cos/1
  Cos/1 -> Product of Elements/1
  Gain1/1 -> ddy/1
  [dy] -> Square/1, Sign/1
  Square/1 -> Gain/1
  Sign/1 -> Product/2
  Gain/1 -> Product/1
  Product/1 -> Add1/2
  Gain2/1 -> y_thrust/1

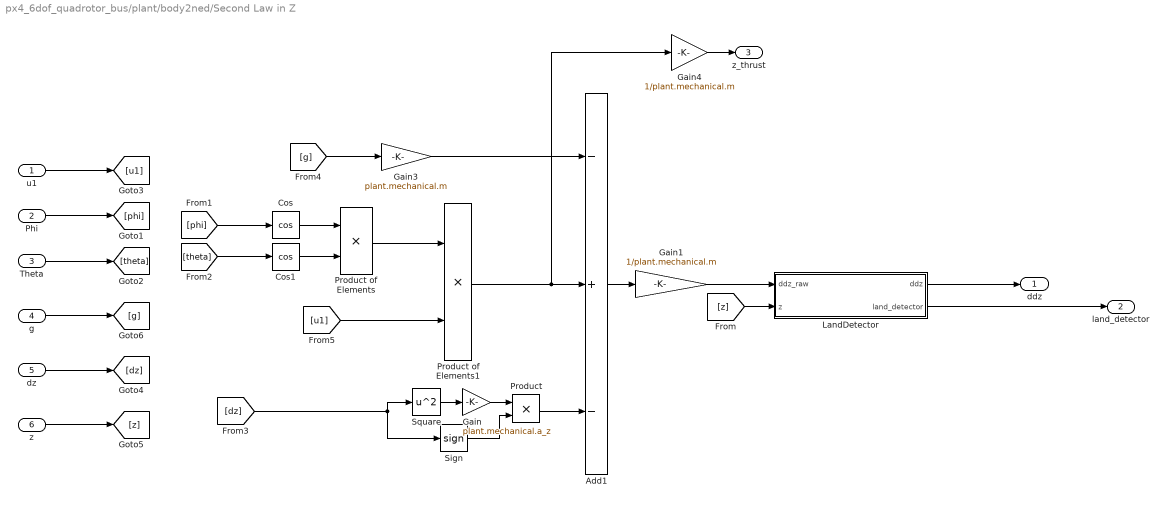
== system px4_6dof_quadrotor_bus/plant/body2ned/Second Law in Z ==
  u1 : Inport
  Phi : Inport  Port=2
  Theta : Inport  Port=3
  g : Inport  Port=4
  dz : Inport  Port=5
  z : Inport  Port=6
  Add1 : Sum  Inputs=-+-
  Cos : Trigonometry  Operator=cos
  Cos1 : Trigonometry  Operator=cos
  Gain : Gain  Gain=plant.mechanical.a_z
  Gain1 : Gain  Gain=1/plant.mechanical.m
  Gain3 : Gain  Gain=plant.mechanical.m
  Gain4 : Gain  Gain=1/plant.mechanical.m
  LandDetector : MATLAB Function  TreatAsAtomicUnit=on
  Product : Product
  Product of Elements : Product
  Product of Elements1 : Product
  Sign : Signum
  Square : Math  Operator=square  SaturateOnIntegerOverflow=on
  ddz : Outport
  land_detector : Outport  Port=2
  z_thrust : Outport  Port=3
  wires:
  Product of Elements1/1 -> Gain4/1, Add1/2
  [u1] -> Product of Elements1/2
  Add1/1 -> Gain1/1
  g/1 -> [g]
  Phi/1 -> [phi]
  Theta/1 -> [theta]
  u1/1 -> [u1]
  dz/1 -> [dz]
  Product of Elements/1 -> Product of Elements1/1
  Cos/1 -> Product of Elements/1
  [phi] -> Cos/1
  Cos1/1 -> Product of Elements/2
  [theta] -> Cos1/1
  Gain1/1 -> LandDetector/1(ddz_raw)
  Square/1 -> Gain/1
  Sign/1 -> Product/2
  Gain/1 -> Product/1
  Product/1 -> Add1/3
  Gain4/1 -> z_thrust/1
  [g] -> Gain3/1
  Gain3/1 -> Add1/1
  z/1 -> [z]
  [z] -> LandDetector/2(z)
  LandDetector/1(ddz) -> ddz/1
  [dz] -> Sign/1, Square/1
  LandDetector/2(land_detector) -> land_detector/1

== system px4_6dof_quadrotor_bus/plant/control2motors/Current Controller1 ==
  Current_error : Inport
  Discrete-Time Integrator : DiscreteIntegrator  SampleTime=plant.motor.electric_time_sample  ICPrevOutput=DiscIntNeverNeededParam  ICPrevScaledInput=DiscIntNeverNeededParam
  Gain : Gain  Gain=db2mag(65)
  Lag : Subsystem  mask{Beta=10000, Freq=300}
      mask prompts: Beta "Beta ="; Freq "Freq [rad/sec] ="
      mask DialogControl DescTextVar Prompt: Lag controller. Choose the frequency and beta.
      mask Display: disp('Lag')
  Lag1 : Subsystem  Commented=on  mask{Beta=10000, Freq=300}
      mask prompts: Beta "Beta ="; Freq "Freq [rad/sec] ="
      mask DialogControl DescTextVar Prompt: Lag controller. Choose the frequency and beta.
      mask Display: disp('Lag')
  Lead : Subsystem  mask{Phase=60, Freq=2*pi*1000}
      mask prompts: Phase "Phase [deg] ="; Freq "Freq [rad/sec] ="
      mask DialogControl DescTextVar Prompt: First order lead controller. Choose the phase you want and the desired frequency.
      mask Display: disp('Lead')
  Notch : Subsystem  Commented=on  mask{wn=20, wd=20, zn=20, zd=20}
      mask prompts: wn "w_n [rad/sec]"; wd "w_d [rad/sec]"; zn "z_n"; zd "z_d"
      mask DialogControl DescTextVar Prompt: Notch filter
      mask Display: disp('Notch')
  Subsystem1 : Subsystem  Commented=on  mask{Phase=20, Freq=4500}
      mask prompts: Phase "Phase [deg] ="; Freq "Freq [rad/sec] ="
      mask DialogControl DescTextVar Prompt: First order lead controller. Choose the phase you want and the desired frequency.
      mask Display: disp('Lead')
  Voltage_cmd : Outport
  wires:
  Lead/1(Out1) -> Gain/1
  Current_error/1 -> Lag/1(In1)
  Discrete-Time Integrator/1 -> Voltage_cmd/1
  Lag/1(Out1) -> Lead/1(In1)
  Gain/1 -> Discrete-Time Integrator/1

== system px4_6dof_quadrotor_bus/plant/control2motors/Current Controller2 ==
  Current_error : Inport
  Discrete-Time Integrator : DiscreteIntegrator  SampleTime=plant.motor.electric_time_sample  ICPrevOutput=DiscIntNeverNeededParam  ICPrevScaledInput=DiscIntNeverNeededParam
  Gain : Gain  Gain=db2mag(65)
  Lag : Subsystem  mask{Beta=10000, Freq=300}
      mask prompts: Beta "Beta ="; Freq "Freq [rad/sec] ="
      mask DialogControl DescTextVar Prompt: Lag controller. Choose the frequency and beta.
      mask Display: disp('Lag')
  Lag1 : Subsystem  Commented=on  mask{Beta=10000, Freq=300}
      mask prompts: Beta "Beta ="; Freq "Freq [rad/sec] ="
      mask DialogControl DescTextVar Prompt: Lag controller. Choose the frequency and beta.
      mask Display: disp('Lag')
  Lead : Subsystem  mask{Phase=60, Freq=2*pi*1000}
      mask prompts: Phase "Phase [deg] ="; Freq "Freq [rad/sec] ="
      mask DialogControl DescTextVar Prompt: First order lead controller. Choose the phase you want and the desired frequency.
      mask Display: disp('Lead')
  Notch : Subsystem  Commented=on  mask{wn=20, wd=20, zn=20, zd=20}
      mask prompts: wn "w_n [rad/sec]"; wd "w_d [rad/sec]"; zn "z_n"; zd "z_d"
      mask DialogControl DescTextVar Prompt: Notch filter
      mask Display: disp('Notch')
  Subsystem1 : Subsystem  Commented=on  mask{Phase=20, Freq=4500}
      mask prompts: Phase "Phase [deg] ="; Freq "Freq [rad/sec] ="
      mask DialogControl DescTextVar Prompt: First order lead controller. Choose the phase you want and the desired frequency.
      mask Display: disp('Lead')
  Voltage_cmd : Outport
  wires:
  Lead/1(Out1) -> Gain/1
  Current_error/1 -> Lag/1(In1)
  Discrete-Time Integrator/1 -> Voltage_cmd/1
  Lag/1(Out1) -> Lead/1(In1)
  Gain/1 -> Discrete-Time Integrator/1

== system px4_6dof_quadrotor_bus/plant/control2motors/Current Controller3 ==
  Current_error : Inport
  Discrete-Time Integrator : DiscreteIntegrator  SampleTime=plant.motor.electric_time_sample  ICPrevOutput=DiscIntNeverNeededParam  ICPrevScaledInput=DiscIntNeverNeededParam
  Gain : Gain  Gain=db2mag(65)
  Lag : Subsystem  mask{Beta=10000, Freq=300}
      mask prompts: Beta "Beta ="; Freq "Freq [rad/sec] ="
      mask DialogControl DescTextVar Prompt: Lag controller. Choose the frequency and beta.
      mask Display: disp('Lag')
  Lag1 : Subsystem  Commented=on  mask{Beta=10000, Freq=300}
      mask prompts: Beta "Beta ="; Freq "Freq [rad/sec] ="
      mask DialogControl DescTextVar Prompt: Lag controller. Choose the frequency and beta.
      mask Display: disp('Lag')
  Lead : Subsystem  mask{Phase=60, Freq=2*pi*1000}
      mask prompts: Phase "Phase [deg] ="; Freq "Freq [rad/sec] ="
      mask DialogControl DescTextVar Prompt: First order lead controller. Choose the phase you want and the desired frequency.
      mask Display: disp('Lead')
  Notch : Subsystem  Commented=on  mask{wn=20, wd=20, zn=20, zd=20}
      mask prompts: wn "w_n [rad/sec]"; wd "w_d [rad/sec]"; zn "z_n"; zd "z_d"
      mask DialogControl DescTextVar Prompt: Notch filter
      mask Display: disp('Notch')
  Subsystem1 : Subsystem  Commented=on  mask{Phase=20, Freq=4500}
      mask prompts: Phase "Phase [deg] ="; Freq "Freq [rad/sec] ="
      mask DialogControl DescTextVar Prompt: First order lead controller. Choose the phase you want and the desired frequency.
      mask Display: disp('Lead')
  Voltage_cmd : Outport
  wires:
  Lead/1(Out1) -> Gain/1
  Current_error/1 -> Lag/1(In1)
  Discrete-Time Integrator/1 -> Voltage_cmd/1
  Lag/1(Out1) -> Lead/1(In1)
  Gain/1 -> Discrete-Time Integrator/1

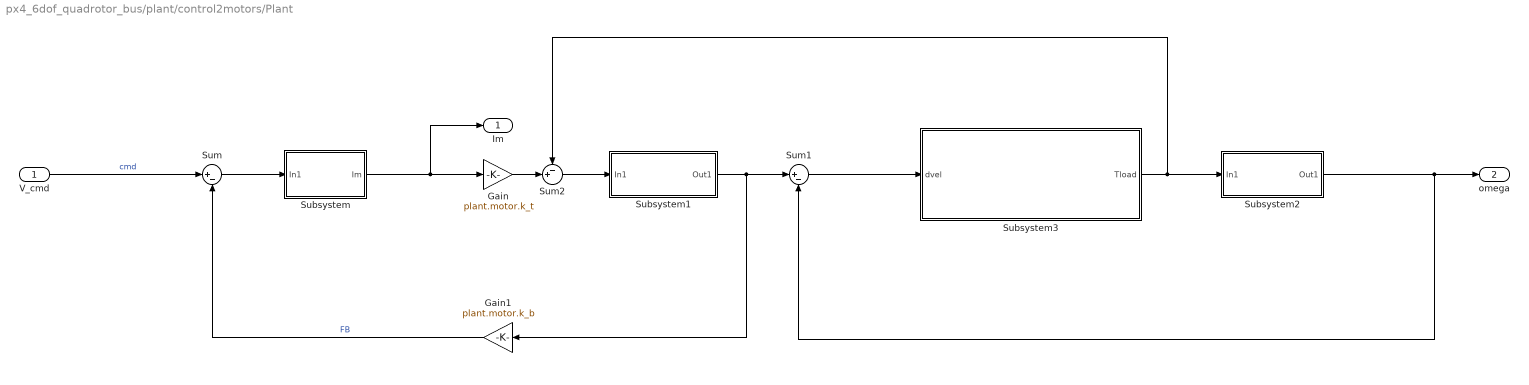
== system px4_6dof_quadrotor_bus/plant/control2motors/Plant ==
  V_cmd : Inport
  Gain : Gain  Gain=plant.motor.k_t
  Gain1 : Gain  Gain=plant.motor.k_b
  Subsystem : Subsystem
      mask Display:
      | disp('1\n')
      | disp('\n----------')
      | disp('\n\n\nLs+R')
  Subsystem1 : Subsystem
      mask Display:
      | disp('1\n')
      | disp('\n----------')
      | disp('\n\n\nJm*s')
  Subsystem2 : Subsystem
      mask Display:
      | disp('1\n')
      | disp('\n----------')
      | disp('\n\n\nJl*s')
  Subsystem3 : Subsystem
  Sum : Sum  Inputs=|+-
  Sum1 : Sum  Inputs=|+-
  Sum2 : Sum  Inputs=-+|
  Im : Outport
  omega : Outport  Port=2
  wires:
  Gain/1 -> Sum2/2
  Sum2/1 -> Subsystem1/1(In1)
  Subsystem3/1(Tload) -> Subsystem2/1(In1), Sum2/1
  Sum1/1 -> Subsystem3/1(dvel)
  Subsystem1/1(Out1) -> Gain1/1, Sum1/1
  Gain1/1 -> Sum/2  "FB"
  V_cmd/1 -> Sum/1  "cmd"
  Sum/1 -> Subsystem/1(In1)
  Subsystem2/1(Out1) -> omega/1, Sum1/2
  Subsystem/1(Im) -> Im/1, Gain/1

== system px4_6dof_quadrotor_bus/plant/control2motors/Plant1 ==
  V_cmd : Inport
  Gain : Gain  Gain=plant.motor.k_t
  Gain1 : Gain  Gain=plant.motor.k_b
  Subsystem : Subsystem
      mask Display:
      | disp('1\n')
      | disp('\n----------')
      | disp('\n\n\nLs+R')
  Subsystem1 : Subsystem
      mask Display:
      | disp('1\n')
      | disp('\n----------')
      | disp('\n\n\nJm*s')
  Subsystem2 : Subsystem
      mask Display:
      | disp('1\n')
      | disp('\n----------')
      | disp('\n\n\nJl*s')
  Subsystem3 : Subsystem
  Sum : Sum  Inputs=|+-
  Sum1 : Sum  Inputs=|+-
  Sum2 : Sum  Inputs=-+|
  Im : Outport
  omega : Outport  Port=2
  wires:
  Gain/1 -> Sum2/2
  Sum2/1 -> Subsystem1/1(In1)
  Sum1/1 -> Subsystem3/1(dvel)
  Subsystem1/1(Out1) -> Gain1/1, Sum1/1
  Gain1/1 -> Sum/2  "FB"
  V_cmd/1 -> Sum/1  "cmd"
  Sum/1 -> Subsystem/1(In1)
  Subsystem2/1(Out1) -> omega/1, Sum1/2
  Subsystem/1(Im) -> Im/1, Gain/1
  Subsystem3/1(Tload) -> Subsystem2/1(In1), Sum2/1

== system px4_6dof_quadrotor_bus/plant/control2motors/Plant2 ==
  V_cmd : Inport
  Gain : Gain  Gain=plant.motor.k_t
  Gain1 : Gain  Gain=plant.motor.k_b
  Subsystem : Subsystem
      mask Display:
      | disp('1\n')
      | disp('\n----------')
      | disp('\n\n\nLs+R')
  Subsystem1 : Subsystem
      mask Display:
      | disp('1\n')
      | disp('\n----------')
      | disp('\n\n\nJm*s')
  Subsystem2 : Subsystem
      mask Display:
      | disp('1\n')
      | disp('\n----------')
      | disp('\n\n\nJl*s')
  Subsystem3 : Subsystem
  Sum : Sum  Inputs=|+-
  Sum1 : Sum  Inputs=|+-
  Sum2 : Sum  Inputs=-+|
  Im : Outport
  omega : Outport  Port=2
  wires:
  Gain/1 -> Sum2/2
  Sum2/1 -> Subsystem1/1(In1)
  Subsystem3/1(Tload) -> Subsystem2/1(In1), Sum2/1
  Sum1/1 -> Subsystem3/1(dvel)
  Subsystem1/1(Out1) -> Gain1/1, Sum1/1
  Gain1/1 -> Sum/2  "FB"
  V_cmd/1 -> Sum/1  "cmd"
  Sum/1 -> Subsystem/1(In1)
  Subsystem2/1(Out1) -> omega/1, Sum1/2
  Subsystem/1(Im) -> Im/1, Gain/1

== system px4_6dof_quadrotor_bus/plant/control2motors/Plant3 ==
  V_cmd : Inport
  Gain : Gain  Gain=plant.motor.k_t
  Gain1 : Gain  Gain=plant.motor.k_b
  Subsystem : Subsystem
      mask Display:
      | disp('1\n')
      | disp('\n----------')
      | disp('\n\n\nLs+R')
  Subsystem1 : Subsystem
      mask Display:
      | disp('1\n')
      | disp('\n----------')
      | disp('\n\n\nJm*s')
  Subsystem2 : Subsystem
      mask Display:
      | disp('1\n')
      | disp('\n----------')
      | disp('\n\n\nJl*s')
  Subsystem3 : Subsystem
  Sum : Sum  Inputs=|+-
  Sum1 : Sum  Inputs=|+-
  Sum2 : Sum  Inputs=-+|
  Im : Outport
  omega : Outport  Port=2
  wires:
  Gain/1 -> Sum2/2
  Sum2/1 -> Subsystem1/1(In1)
  Subsystem3/1(Tload) -> Subsystem2/1(In1), Sum2/1
  Sum1/1 -> Subsystem3/1(dvel)
  Subsystem1/1(Out1) -> Gain1/1, Sum1/1
  Gain1/1 -> Sum/2  "FB"
  V_cmd/1 -> Sum/1  "cmd"
  Sum/1 -> Subsystem/1(In1)
  Subsystem2/1(Out1) -> omega/1, Sum1/2
  Subsystem/1(Im) -> Im/1, Gain/1

== system px4_6dof_quadrotor_bus/plant/control2motors/Velocity Controller ==
  Velocity_error : Inport
  Gain : Gain  Gain=db2mag(-42)
  Lag1 : Subsystem  Commented=on  mask{Beta=10000, Freq=300}
      mask prompts: Beta "Beta ="; Freq "Freq [rad/sec] ="
      mask DialogControl DescTextVar Prompt: Lag controller. Choose the frequency and beta.
      mask Display: disp('Lag')
  Notch : Subsystem  Commented=on  mask{wn=20, wd=20, zn=20, zd=20}
      mask prompts: wn "w_n [rad/sec]"; wd "w_d [rad/sec]"; zn "z_n"; zd "z_d"
      mask DialogControl DescTextVar Prompt: Notch filter
      mask Display: disp('Notch')
  Subsystem1 : Subsystem  Commented=on  mask{Phase=20, Freq=4500}
      mask prompts: Phase "Phase [deg] ="; Freq "Freq [rad/sec] ="
      mask DialogControl DescTextVar Prompt: First order lead controller. Choose the phase you want and the desired frequency.
      mask Display: disp('Lead')
  Current_cmd : Outport
  wires:
  Gain/1 -> Current_cmd/1
  Velocity_error/1 -> Gain/1

== system px4_6dof_quadrotor_bus/plant/control2motors/Velocity Controller1 ==
  Velocity_error : Inport
  Gain : Gain  Gain=db2mag(-42)
  Lag1 : Subsystem  Commented=on  mask{Beta=10000, Freq=300}
      mask prompts: Beta "Beta ="; Freq "Freq [rad/sec] ="
      mask DialogControl DescTextVar Prompt: Lag controller. Choose the frequency and beta.
      mask Display: disp('Lag')
  Notch : Subsystem  Commented=on  mask{wn=20, wd=20, zn=20, zd=20}
      mask prompts: wn "w_n [rad/sec]"; wd "w_d [rad/sec]"; zn "z_n"; zd "z_d"
      mask DialogControl DescTextVar Prompt: Notch filter
      mask Display: disp('Notch')
  Subsystem1 : Subsystem  Commented=on  mask{Phase=20, Freq=4500}
      mask prompts: Phase "Phase [deg] ="; Freq "Freq [rad/sec] ="
      mask DialogControl DescTextVar Prompt: First order lead controller. Choose the phase you want and the desired frequency.
      mask Display: disp('Lead')
  Current_cmd : Outport
  wires:
  Gain/1 -> Current_cmd/1
  Velocity_error/1 -> Gain/1

== system px4_6dof_quadrotor_bus/plant/control2motors/Velocity Controller2 ==
  Velocity_error : Inport
  Gain : Gain  Gain=db2mag(-42)
  Lag1 : Subsystem  Commented=on  mask{Beta=10000, Freq=300}
      mask prompts: Beta "Beta ="; Freq "Freq [rad/sec] ="
      mask DialogControl DescTextVar Prompt: Lag controller. Choose the frequency and beta.
      mask Display: disp('Lag')
  Notch : Subsystem  Commented=on  mask{wn=20, wd=20, zn=20, zd=20}
      mask prompts: wn "w_n [rad/sec]"; wd "w_d [rad/sec]"; zn "z_n"; zd "z_d"
      mask DialogControl DescTextVar Prompt: Notch filter
      mask Display: disp('Notch')
  Subsystem1 : Subsystem  Commented=on  mask{Phase=20, Freq=4500}
      mask prompts: Phase "Phase [deg] ="; Freq "Freq [rad/sec] ="
      mask DialogControl DescTextVar Prompt: First order lead controller. Choose the phase you want and the desired frequency.
      mask Display: disp('Lead')
  Current_cmd : Outport
  wires:
  Gain/1 -> Current_cmd/1
  Velocity_error/1 -> Gain/1

== system px4_6dof_quadrotor_bus/plant/control2motors/Velocity Controller3 ==
  Velocity_error : Inport
  Gain : Gain  Gain=db2mag(-42)
  Lag1 : Subsystem  Commented=on  mask{Beta=10000, Freq=300}
      mask prompts: Beta "Beta ="; Freq "Freq [rad/sec] ="
      mask DialogControl DescTextVar Prompt: Lag controller. Choose the frequency and beta.
      mask Display: disp('Lag')
  Notch : Subsystem  Commented=on  mask{wn=20, wd=20, zn=20, zd=20}
      mask prompts: wn "w_n [rad/sec]"; wd "w_d [rad/sec]"; zn "z_n"; zd "z_d"
      mask DialogControl DescTextVar Prompt: Notch filter
      mask Display: disp('Notch')
  Subsystem1 : Subsystem  Commented=on  mask{Phase=20, Freq=4500}
      mask prompts: Phase "Phase [deg] ="; Freq "Freq [rad/sec] ="
      mask DialogControl DescTextVar Prompt: First order lead controller. Choose the phase you want and the desired frequency.
      mask Display: disp('Lead')
  Current_cmd : Outport
  wires:
  Gain/1 -> Current_cmd/1
  Velocity_error/1 -> Gain/1

== system px4_6dof_quadrotor_bus/plant/control2motors/Current Controller1/Lag ==
  In1 : Inport
  LTI System : cstblocks/LTI System  sys=c2d(lag(Freq,Beta),plant.motor.electric_time_sample)  IC=[]
  Out1 : Outport
  wires:
  LTI System/1 -> Out1/1
  In1/1 -> LTI System/1

== system px4_6dof_quadrotor_bus/plant/control2motors/Current Controller1/Lag1 ==
  In1 : Inport
  LTI System : cstblocks/LTI System  sys=lag(Freq,Beta)  IC=[]
  Out1 : Outport
  wires:
  In1/1 -> LTI System/1
  LTI System/1 -> Out1/1

== system px4_6dof_quadrotor_bus/plant/control2motors/Current Controller1/Lead ==
  In1 : Inport
  LTI System : cstblocks/LTI System  sys=c2d(lead(Phase,Freq),plant.motor.electric_time_sample)  IC=[]
  Out1 : Outport
  wires:
  LTI System/1 -> Out1/1
  In1/1 -> LTI System/1

== system px4_6dof_quadrotor_bus/plant/control2motors/Current Controller1/Notch ==
  In1 : Inport
  LTI System : cstblocks/LTI System  sys=notch(wn,wd,zn,zd)  IC=[]
  Out1 : Outport
  wires:
  LTI System/1 -> Out1/1
  In1/1 -> LTI System/1

== system px4_6dof_quadrotor_bus/plant/control2motors/Current Controller1/Subsystem1 ==
  In1 : Inport
  LTI System : cstblocks/LTI System  sys=lead(Phase,Freq)  IC=[]
  Out1 : Outport
  wires:
  In1/1 -> LTI System/1
  LTI System/1 -> Out1/1

== system px4_6dof_quadrotor_bus/plant/control2motors/Current Controller2/Lag ==
  In1 : Inport
  LTI System : cstblocks/LTI System  sys=c2d(lag(Freq,Beta),plant.motor.electric_time_sample)  IC=[]
  Out1 : Outport
  wires:
  LTI System/1 -> Out1/1
  In1/1 -> LTI System/1

== system px4_6dof_quadrotor_bus/plant/control2motors/Current Controller2/Lag1 ==
  In1 : Inport
  LTI System : cstblocks/LTI System  sys=lag(Freq,Beta)  IC=[]
  Out1 : Outport
  wires:
  In1/1 -> LTI System/1
  LTI System/1 -> Out1/1

== system px4_6dof_quadrotor_bus/plant/control2motors/Current Controller2/Lead ==
  In1 : Inport
  LTI System : cstblocks/LTI System  sys=c2d(lead(Phase,Freq),plant.motor.electric_time_sample)  IC=[]
  Out1 : Outport
  wires:
  LTI System/1 -> Out1/1
  In1/1 -> LTI System/1

== system px4_6dof_quadrotor_bus/plant/control2motors/Current Controller2/Notch ==
  In1 : Inport
  LTI System : cstblocks/LTI System  sys=notch(wn,wd,zn,zd)  IC=[]
  Out1 : Outport
  wires:
  LTI System/1 -> Out1/1
  In1/1 -> LTI System/1

== system px4_6dof_quadrotor_bus/plant/control2motors/Current Controller2/Subsystem1 ==
  In1 : Inport
  LTI System : cstblocks/LTI System  sys=lead(Phase,Freq)  IC=[]
  Out1 : Outport
  wires:
  In1/1 -> LTI System/1
  LTI System/1 -> Out1/1

== system px4_6dof_quadrotor_bus/plant/control2motors/Current Controller3/Lag ==
  In1 : Inport
  LTI System : cstblocks/LTI System  sys=c2d(lag(Freq,Beta),plant.motor.electric_time_sample)  IC=[]
  Out1 : Outport
  wires:
  LTI System/1 -> Out1/1
  In1/1 -> LTI System/1

== system px4_6dof_quadrotor_bus/plant/control2motors/Current Controller3/Lag1 ==
  In1 : Inport
  LTI System : cstblocks/LTI System  sys=lag(Freq,Beta)  IC=[]
  Out1 : Outport
  wires:
  In1/1 -> LTI System/1
  LTI System/1 -> Out1/1

== system px4_6dof_quadrotor_bus/plant/control2motors/Current Controller3/Lead ==
  In1 : Inport
  LTI System : cstblocks/LTI System  sys=c2d(lead(Phase,Freq),plant.motor.electric_time_sample)  IC=[]
  Out1 : Outport
  wires:
  LTI System/1 -> Out1/1
  In1/1 -> LTI System/1

== system px4_6dof_quadrotor_bus/plant/control2motors/Current Controller3/Notch ==
  In1 : Inport
  LTI System : cstblocks/LTI System  sys=notch(wn,wd,zn,zd)  IC=[]
  Out1 : Outport
  wires:
  LTI System/1 -> Out1/1
  In1/1 -> LTI System/1

== system px4_6dof_quadrotor_bus/plant/control2motors/Current Controller3/Subsystem1 ==
  In1 : Inport
  LTI System : cstblocks/LTI System  sys=lead(Phase,Freq)  IC=[]
  Out1 : Outport
  wires:
  In1/1 -> LTI System/1
  LTI System/1 -> Out1/1

== system px4_6dof_quadrotor_bus/plant/control2motors/Plant/Subsystem ==
  In1 : Inport
  Discrete-Time Integrator : DiscreteIntegrator  SampleTime=-1  ICPrevOutput=DiscIntNeverNeededParam  ICPrevScaledInput=DiscIntNeverNeededParam
  Gain : Gain  Gain=plant.motor.r
  Gain1 : Gain  Gain=1/plant.motor.l
  Sum : Sum  Inputs=|+-
  Im : Outport
  wires:
  Gain/1 -> Sum/2
  Gain1/1 -> Discrete-Time Integrator/1
  Discrete-Time Integrator/1 -> Im/1, Gain/1
  Sum/1 -> Gain1/1
  In1/1 -> Sum/1

== system px4_6dof_quadrotor_bus/plant/control2motors/Plant/Subsystem1 ==
  In1 : Inport
  Discrete-Time Integrator : DiscreteIntegrator  SampleTime=plant.motor.electric_time_sample  ICPrevOutput=DiscIntNeverNeededParam  ICPrevScaledInput=DiscIntNeverNeededParam
  Gain : Gain  Gain=1/plant.motor.j_m
  Out1 : Outport
  wires:
  Gain/1 -> Out1/1
  Discrete-Time Integrator/1 -> Gain/1
  In1/1 -> Discrete-Time Integrator/1

== system px4_6dof_quadrotor_bus/plant/control2motors/Plant/Subsystem2 ==
  In1 : Inport
  Discrete-Time Integrator : DiscreteIntegrator  SampleTime=plant.motor.electric_time_sample  ICPrevOutput=DiscIntNeverNeededParam  ICPrevScaledInput=DiscIntNeverNeededParam
  Gain : Gain  Gain=1/plant.motor.j_l
  Out1 : Outport
  wires:
  Gain/1 -> Out1/1
  In1/1 -> Discrete-Time Integrator/1
  Discrete-Time Integrator/1 -> Gain/1

== system px4_6dof_quadrotor_bus/plant/control2motors/Plant/Subsystem3 ==
  dvel : Inport
  Add : Sum
  Discrete-Time Integrator : DiscreteIntegrator  SampleTime=plant.motor.electric_time_sample  ICPrevOutput=DiscIntNeverNeededParam  ICPrevScaledInput=DiscIntNeverNeededParam
  Gain2 : Gain  Gain=plant.motor.k_v
  Gain5 : Gain  Gain=plant.motor.k_k
  Tload : Outport
  wires:
  Add/1 -> Tload/1
  Gain2/1 -> Add/1
  Gain5/1 -> Add/2
  dvel/1 -> Discrete-Time Integrator/1, Gain2/1
  Discrete-Time Integrator/1 -> Gain5/1
